simulink model "Simulation"  (R2026a)
settings: Solver=FixedStepAuto  StopTime=35  FixedStep=0.001  MaxStep=0.01  RelTol=1e-6
values from neighbouring files (symbols this model uses):
  a_max = 9.364072394    [params.m]    (also in scurve_test.m = 9.364)
  eta = 0.85    [params.m]
  j_max = 93.64072394    [params.m]
  K_aff = 0    [params.m]
  k_e = (V_max - (I_rated * R_m)) / omega_m    (= 0.0320704010623)    [params.m]
  k_t = tau_m / I_rated    (= 0.0381971863421)    [params.m]
  K_vff = 0    [params.m]
  L_m = 0.00147261    [params.m]
  N_total = N_gear * N_belt    (= 70)    [params.m]    (also in setup.m)
  q_final = 2*pi    (= 6.28318530718)    [params.m]
  q_init = 0    [params.m]
  R_m = 1.53982909    [params.m]
  v_max = 8.97597901    [params.m]
undefined symbols (not defined in the file or in its folder): X, Y, Z
libraries: sm_lib x16, nesl_utility x7, slpidlib x1
settings Model: Creator=thadzy  LastModifiedBy=thadzy
settings SimscapeCC: SimscapeNominalValues="[{\"value\":\"1\",\"unit\":\"A\"},{\"value\":\"1\",\"unit\":\"bar\"},{\"value\":\"1\",\"unit\":\"cm^2\"},{\"value\":\"1\",\"unit\":\"cm^3/s\"},{\"value\":\"1\",\"unit\":\"kJ/kg\"},{\"value\":\"1\",\"unit\":\"kW\"},{\"value\":\"1\",\"unit\":\"l\"},{\"value\":\"1\",\"unit\":\"N\"},{\"value\":\"1\",\"unit\":\"N*m\"},{\"value\":\"1\",\"unit\":\"V\"}]"  SimscapeLogType=none  SimscapeLogDataHistory=5000.0

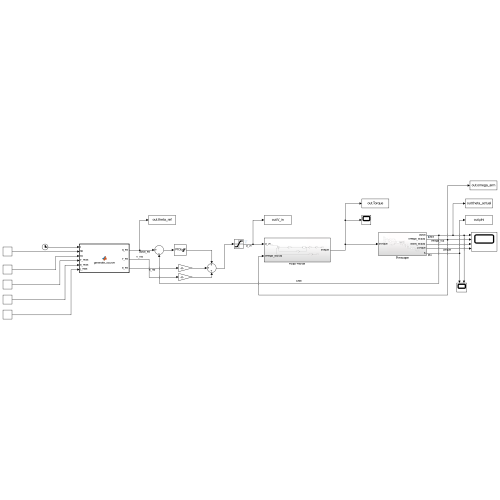
[thumbnail: Simulink's stored preview of the top-level diagram]
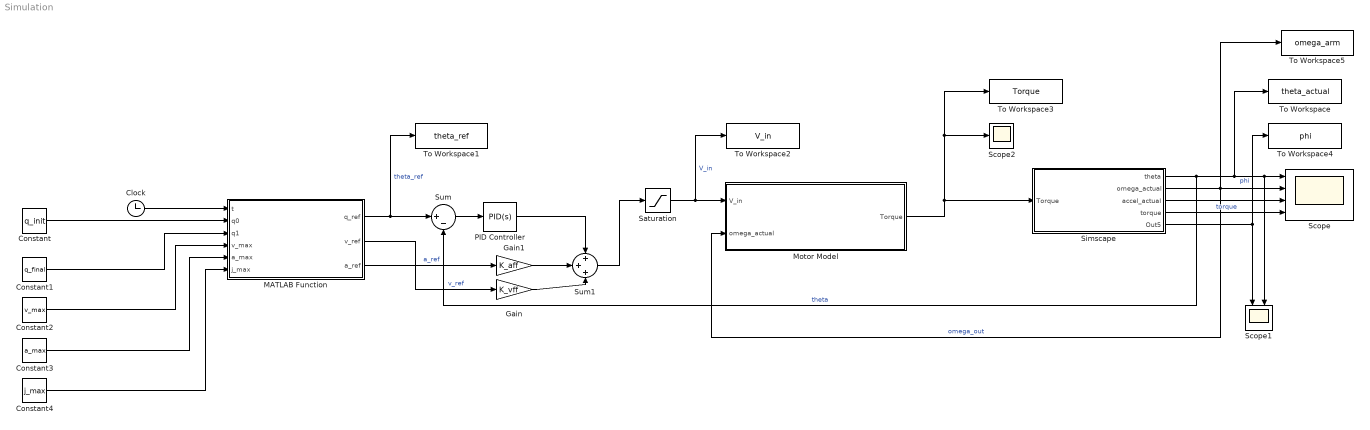
== system Simulation ==
  Clock : Clock
  Constant : Constant  Value=q_init
  Constant1 : Constant  Value=q_final
  Constant2 : Constant  Value=v_max
  Constant3 : Constant  Value=a_max
  Constant4 : Constant  Value=j_max
  Gain : Gain  Gain=K_vff
  Gain1 : Gain  Gain=K_aff
  MATLAB Function : MATLAB Function  TreatAsAtomicUnit=on
  Motor Model : Subsystem
  PID Controller : slpidlib/PID Controller  Controller=PID  Form=Parallel  TimeDomain=Continuous-time  UseExternalTs=off  SampleTime=-1  IntegratorMethod=Forward Euler  FilterMethod=Forward Euler  ControllerParametersSource=internal  P=1  I=0  UseKiTs=off  D=0.5  UseExternalDerivativeSource=off  N=200  UseFilter=on  TunerSelectOption=Transfer Function Based (PID Tuner App)  InitialConditionSource=internal  InitialConditionForIntegrator=0  InitialConditionForFilter=0  DifferentiatorICPrevScaledInput=0  ExternalReset=none  TrackingMode=off  Kt=1  LimitOutput=on  SatLimitsSource=internal  UpperSaturationLimit=24  LowerSaturationLimit=-24  LinearizeAsGain=on  AntiWindupMode=clamping  Kb=1  LimitIntegrator=off  UpperIntegratorSaturationLimit=inf  LowerIntegratorSaturationLimit=-inf  POutMin=[]  POutMax=[]  IOutMin=[]  IOutMax=[]  DOutMin=[]  DOutMax=[]  NOutMin=[]  NOutMax=[]  SumOutMin=[]  SumOutMax=[]  SaturationOutMin=[]  SaturationOutMax=[]  PParamMin=[]  PParamMax=[]  IParamMin=[]  IParamMax=[]  DParamMin=[]  DParamMax=[]  NParamMin=[]  NParamMax=[]  KbParamMin=[]  KbParamMax=[]  KtParamMin=[]  KtParamMax=[]  KbOutMin=[]  KbOutMax=[]  KtOutMin=[]  KtOutMax=[]  IntegratorOutMin=[]  IntegratorOutMax=[]  FilterOutMin=[]  FilterOutMax=[]  SumI1OutMin=[]  SumI1OutMax=[]  SumI2OutMin=[]  SumI2OutMax=[]  SumI3OutMin=[]  SumI3OutMax=[]  SumI4OutMin=[]  SumI4OutMax=[]  SumDOutMin=[]  SumDOutMax=[]  DifferentiatorOutMin=[]  DifferentiatorOutMax=[]  FilterDiffOutCoefMin=[]  FilterDiffOutCoefMax=[]  ReciprocalOutMin=[]  ReciprocalOutMax=[]  SumDenOutMin=[]  SumDenOutMax=[]  SumNumOutMin=[]  SumNumOutMax=[]  DivideOutMin=[]  DivideOutMax=[]  UdiffTsProdOutMin=[]  UdiffTsProdOutMax=[]  NTsProdOutMin=[]  NTsProdOutMax=[]  UintegralTsProdOutMin=[]  UintegralTsProdOutMax=[]  UngainTsProdOutMin=[]  UngainTsProdOutMax=[]  ClampingZeroOutDataTypeStr=Inherit: Inherit via back propagation  ClampingZeroOutMin=[]  ClampingZeroOutMax=[]  FilterDenConstantOutDataTypeStr=Inherit: Inherit via back propagation  FilterDenConstantOutMin=[]  FilterDenConstantOutMax=[]  PCopyOutDataTypeStr=Inherit: Inherit via back propagation  PCopyOutMin=[]  PCopyOutMax=[]  NCopyOutDataTypeStr=Inherit: Inherit via back propagation  NCopyOutMin=[]  NCopyOutMax=[]  IntegratorContinuousStateAttributes=''  IntegratorStateMustResolveToSignalObject=off  IntegratorRTWStateStorageClass=Auto  FilterContinuousStateAttributes=''  FilterStateMustResolveToSignalObject=off  FilterRTWStateStorageClass=Auto  ParallelPVariant=InternalParameters  IdealPVariant=Disabled  IVariant=InternalParameters  DVariant=InternalParameters  IntegratorVariant=Continuous  SatVariant=Enabled  AWVariant=ContClampingParallel  PCopyVariant=Disabled  TRVariant=Disabled  FdbkBlocksVariant=Forward  IdealPFdbkVariant=Disabled  SatFdbkVariant=Disabled  DerivativeFilterVariant=ContFilter  NVariant=InternalParameters  NCopyVariant=Disabled  FilterICVariant=InternalICsFilter  IntegratorICVariant=InternalICs  ExternalResetVariant=Disabled  TRSumVariant=Passthrough  SumFdbkVariant=Disabled  SumVariant=Sum_PID  TsampFilterVariant=InternalTs  TsampNgainVariant=Passthrough  TsampIntegralVariant=Disabled_SignalSpec  ExternalSaturationOutDataTypeStr=Inherit: Same as second input  DerivativeSourceVariant=ErrorSignal  PreIntVariant=InternalPreInt
  Saturation : Saturate  UpperLimit=24  LowerLimit=-24
  Scope : Scope  NumInputPorts=4
      settings: ActiveDisplayYMinimum=-23.989705041384052  ActiveDisplayYMaximum=22.744388235078567
  Scope1 : Scope  NumInputPorts=2
      settings: ActiveDisplayYMinimum=-16.623926963766117  ActiveDisplayYMaximum=10.381312120570854
  Scope2 : Scope
      settings: ActiveDisplayYMinimum=-0.24844726502323963  ActiveDisplayYMaximum=0.27894907226779375  DataLoggingVariableName=ScopeData2
  Simscape : Subsystem
  Sum : Sum  Inputs=|+-
  Sum1 : Sum  Inputs=+++
  To Workspace : ToWorkspace  VariableName=theta_actual  SaveFormat=Timeseries  SampleTime=-1
  To Workspace1 : ToWorkspace  VariableName=theta_ref  SaveFormat=Timeseries  SampleTime=-1
  To Workspace2 : ToWorkspace  VariableName=V_in  SaveFormat=Timeseries  SampleTime=-1
  To Workspace3 : ToWorkspace  VariableName=Torque  SaveFormat=Timeseries  SampleTime=-1
  To Workspace4 : ToWorkspace  VariableName=phi  SaveFormat=Timeseries  SampleTime=-1
  To Workspace5 : ToWorkspace  VariableName=omega_arm  SaveFormat=Timeseries  SampleTime=-1
  wires:
  Simscape/1(theta) -> To Workspace/1, Scope1/2, Scope/1, Sum/2  "theta"
  Simscape/2(omega_actual) -> To Workspace5/1, Scope/2, Motor Model/2(omega_actual)  "omega_out"
  Simscape/3(accel_actual) -> Scope/3
  Simscape/4(torque) -> Scope/4  "torque"
  Simscape/5(Out5) -> To Workspace4/1, Scope1/1  "phi"
  Motor Model/1(Torque) -> To Workspace3/1, Scope2/1, Simscape/1(Torque)
  Clock/1 -> MATLAB Function/1(t)
  MATLAB Function/1(q_ref) -> To Workspace1/1, Sum/1  "theta_ref"
  Constant/1 -> MATLAB Function/2(q0)
  Constant1/1 -> MATLAB Function/3(q1)
  Constant2/1 -> MATLAB Function/4(v_max)
  Constant3/1 -> MATLAB Function/5(a_max)
  Constant4/1 -> MATLAB Function/6(j_max)
  Sum/1 -> PID Controller/1
  MATLAB Function/2(v_ref) -> Gain/1  "v_ref"
  MATLAB Function/3(a_ref) -> Gain1/1  "a_ref"
  PID Controller/1 -> Sum1/1
  Gain1/1 -> Sum1/2
  Gain/1 -> Sum1/3
  Sum1/1 -> Saturation/1
  Saturation/1 -> To Workspace2/1, Motor Model/1(V_in)  "V_in"

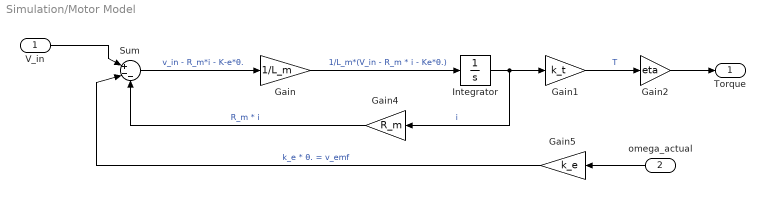
== system Simulation/Motor Model ==
  V_in : Inport
  omega_actual : Inport  Port=2
  Gain : Gain  Gain=1/L_m
  Gain1 : Gain  Gain=k_t
  Gain2 : Gain  Gain=eta
  Gain4 : Gain  Gain=R_m
  Gain5 : Gain  Gain=k_e
  Integrator : Integrator
  Sum : Sum  Inputs=|+--
  Torque : Outport
  wires:
  Gain/1 -> Integrator/1  "1/L_m*(V_in - R_m * i - Ke*θ.)"
  Gain5/1 -> Sum/2  "k_e * θ. = v_emf"
  Integrator/1 -> Gain4/1, Gain1/1  "i"
  V_in/1 -> Sum/1
  Sum/1 -> Gain/1  "v_in - R_m*i - K-e*θ."
  Gain4/1 -> Sum/3  "R_m * i"
  omega_actual/1 -> Gain5/1
  Gain1/1 -> Gain2/1  "T"
  Gain2/1 -> Torque/1

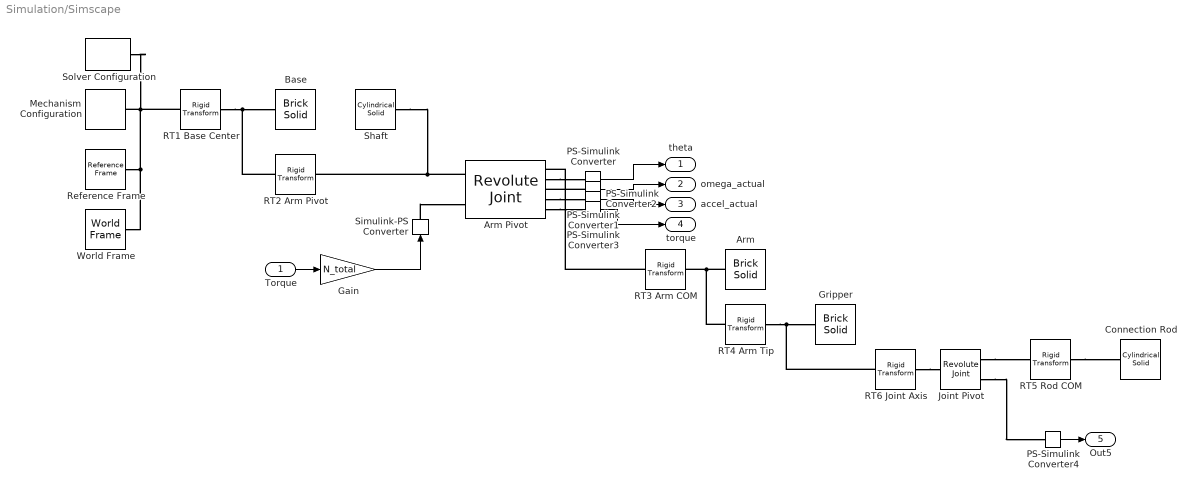
== system Simulation/Simscape ==
  Torque : Inport
  Arm : sm_lib/Body Elements/Brick Solid  BrickDimensions=[0.5 0.025 0.025]  BrickDimensionsUnits=m  ExportEntireGeometry=off  InertiaType=Custom  BasedOnType=Density  Density=2621  DensityUnits=kg/m^3  Mass=0.75357  MassUnits=kg  CenterOfMass=[0 0 0]  CenterOfMassUnits=m  MomentsOfInertia=[0.013479, 0.000131, 0.013479]  MomentsOfInertiaUnits=kg*m^2  ProductsOfInertia=[0, 0, -9.26e-6]  ProductsOfInertiaUnits=kg*m^2  GraphicType=FromGeometry  MarkerShape=Sphere  MarkerSize=10  GraphicVisPropType=SimpleVisualProperties  GraphicDiffuseColor=[0.4941 0.4941 0.502]  GraphicOpacity=1  GraphicSpecularColor=[0.5 0.5 0.5 1.0]  GraphicAmbientColor=[0.15 0.15 0.15 1.0]  GraphicEmissiveColor=[0.0 0.0 0.0 1.0]  GraphicShininess=75  DoExposeReferenceFrame=on  SerializedFrames=<Frames/>
  Arm Pivot : sm_lib/Joints/Revolute Joint  JointMode=Normal  CompositeWrenchDir=FollowerOnBase  CompositeWrenchFrame=BaseFrame  SenseConstraintForce=off  SenseConstraintTorque=off  SenseTotalForce=off  SenseTotalTorque=off  PositionTargetSpecify=off  PositionTargetPriority=High  PositionTargetValue=0  PositionTargetValueUnits=deg  VelocityTargetSpecify=off  VelocityTargetPriority=High  VelocityTargetValue=0  VelocityTargetValueUnits=deg/s  EquilibriumPosition=0  EquilibriumPositionUnits=deg  SpringStiffness=0  SpringStiffnessUnits=N*m/deg  DampingCoefficient=B_arm  DampingCoefficientUnits=N*m/(rad/s)  LowerLimitSpecify=off  LowerLimitBound=-90  LowerLimitBoundUnits=deg  LowerLimitStiffness=1e4  LowerLimitStiffnessUnits=N*m/deg  LowerLimitDamping=10  LowerLimitDampingUnits=N*m/(deg/s)  LowerLimitTransitionRegionWidth=0.1  LowerLimitTransitionRegionWidthUnits=deg  UpperLimitSpecify=off  UpperLimitBound=90  UpperLimitBoundUnits=deg  UpperLimitStiffness=1e4  UpperLimitStiffnessUnits=N*m/deg  UpperLimitDamping=10  UpperLimitDampingUnits=N*m/(deg/s)  UpperLimitTransitionRegionWidth=0.1  UpperLimitTransitionRegionWidthUnits=deg  TorqueActuationMode=InputTorque  MotionActuationMode=ComputedMotion  SensePosition=on  SenseVelocity=on  SenseAcceleration=on  SenseTorqueForce=on  SenseLowerLimitTorqueForce=off  SenseUpperLimitTorqueForce=off
  Base : sm_lib/Body Elements/Brick Solid  BrickDimensions=[0.16 0.16 0.15]  BrickDimensionsUnits=m  ExportEntireGeometry=off  InertiaType=CalculateFromGeometry  BasedOnType=Density  Density=2700  DensityUnits=kg/m^3  Mass=1  MassUnits=kg  CenterOfMass=[0 0 0]  CenterOfMassUnits=m  MomentsOfInertia=[1 1 1]  MomentsOfInertiaUnits=kg*m^2  ProductsOfInertia=[0 0 0]  ProductsOfInertiaUnits=kg*m^2  GraphicType=FromGeometry  MarkerShape=Sphere  MarkerSize=10  GraphicVisPropType=SimpleVisualProperties  GraphicDiffuseColor=[0.02745 0 1]  GraphicOpacity=1  GraphicSpecularColor=[0.5 0.5 0.5 1.0]  GraphicAmbientColor=[0.15 0.15 0.15 1.0]  GraphicEmissiveColor=[0.0 0.0 0.0 1.0]  GraphicShininess=75  DoExposeReferenceFrame=on  SerializedFrames=<Frames/>
  Connection Rod : sm_lib/Body Elements/Cylindrical Solid  CylinderRadius=0.005  CylinderRadiusUnits=m  CylinderLength=0.1  CylinderLengthUnits=m  ExportEntireGeometry=off  InertiaType=Custom  BasedOnType=Density  Density=7850  DensityUnits=kg/m^3  Mass=0.16408  MassUnits=kg  CenterOfMass=[0 0 0]  CenterOfMassUnits=m  MomentsOfInertia=[0.000169, 0.000152, 2.42e-5]  MomentsOfInertiaUnits=kg*m^2  ProductsOfInertia=[0 0 0]  ProductsOfInertiaUnits=kg*m^2  GraphicType=FromGeometry  MarkerShape=Sphere  MarkerSize=10  GraphicVisPropType=SimpleVisualProperties  GraphicDiffuseColor=[1 0 0.02745]  GraphicOpacity=1  GraphicSpecularColor=[0.5 0.5 0.5 1.0]  GraphicAmbientColor=[0.15 0.15 0.15 1.0]  GraphicEmissiveColor=[0.0 0.0 0.0 1.0]  GraphicShininess=75  DoExposeReferenceFrame=on  SerializedFrames=<Frames/>
  Gain : Gain  Gain=N_total
  Gripper : sm_lib/Body Elements/Brick Solid  BrickDimensions=[0.04 0.04 0.04]  BrickDimensionsUnits=m  ExportEntireGeometry=off  InertiaType=Custom  BasedOnType=Density  Density=1000  DensityUnits=kg/m^3  Mass=0.73897  MassUnits=kg  CenterOfMass=[0 0 0]  CenterOfMassUnits=m  MomentsOfInertia=[0.001819, 0.001273, 0.000760]  MomentsOfInertiaUnits=kg*m^2  ProductsOfInertia=[-8.41e-5, -6.54e-6, 9.06e-7]  ProductsOfInertiaUnits=kg*m^2  GraphicType=FromGeometry  MarkerShape=Sphere  MarkerSize=10  GraphicVisPropType=SimpleVisualProperties  GraphicDiffuseColor=[0.0902 1 0]  GraphicOpacity=1  GraphicSpecularColor=[0.5 0.5 0.5 1.0]  GraphicAmbientColor=[0.15 0.15 0.15 1.0]  GraphicEmissiveColor=[0.0 0.0 0.0 1.0]  GraphicShininess=75  DoExposeReferenceFrame=on  SerializedFrames=<Frames/>
  Joint Pivot : sm_lib/Joints/Revolute Joint  JointMode=Normal  CompositeWrenchDir=FollowerOnBase  CompositeWrenchFrame=BaseFrame  SenseConstraintForce=off  SenseConstraintTorque=off  SenseTotalForce=off  SenseTotalTorque=off  PositionTargetSpecify=off  PositionTargetPriority=High  PositionTargetValue=20  PositionTargetValueUnits=deg  VelocityTargetSpecify=off  VelocityTargetPriority=High  VelocityTargetValue=0  VelocityTargetValueUnits=deg/s  EquilibriumPosition=0  EquilibriumPositionUnits=deg  SpringStiffness=0  SpringStiffnessUnits=N*m/deg  DampingCoefficient=0.0006712  DampingCoefficientUnits=N*m/(rad/s)  LowerLimitSpecify=off  LowerLimitBound=-90  LowerLimitBoundUnits=deg  LowerLimitStiffness=1e4  LowerLimitStiffnessUnits=N*m/deg  LowerLimitDamping=10  LowerLimitDampingUnits=N*m/(deg/s)  LowerLimitTransitionRegionWidth=0.1  LowerLimitTransitionRegionWidthUnits=deg  UpperLimitSpecify=off  UpperLimitBound=90  UpperLimitBoundUnits=deg  UpperLimitStiffness=1e4  UpperLimitStiffnessUnits=N*m/deg  UpperLimitDamping=10  UpperLimitDampingUnits=N*m/(deg/s)  UpperLimitTransitionRegionWidth=0.1  UpperLimitTransitionRegionWidthUnits=deg  TorqueActuationMode=NoTorque  MotionActuationMode=ComputedMotion  SensePosition=on  SenseVelocity=off  SenseAcceleration=off  SenseTorqueForce=off  SenseLowerLimitTorqueForce=off  SenseUpperLimitTorqueForce=off
  Mechanism Configuration : sm_lib/Utilities/Mechanism Configuration  UniformGravity=Constant  GravityVector=[0 0 -9.80665]  GravityVectorUnits=m/s^2  LinearizationDelta=0.001  JointModeTransitionNonlinearIterations=2
  PS-Simulink Converter : nesl_utility/PS-Simulink Converter  PhysicalDomain=network_engine_domain  SubClassName=ps_output  LeftPortType=input  RightPortType=output  PseudoPeriodic=off  Frequencies=[]  VectorFormat=inherit  Unit=rad  AffineConversion=off
  PS-Simulink Converter1 : nesl_utility/PS-Simulink Converter  PhysicalDomain=network_engine_domain  SubClassName=ps_output  LeftPortType=input  RightPortType=output  PseudoPeriodic=off  Frequencies=[]  VectorFormat=inherit  Unit=rad/s  AffineConversion=off
  PS-Simulink Converter2 : nesl_utility/PS-Simulink Converter  PhysicalDomain=network_engine_domain  SubClassName=ps_output  LeftPortType=input  RightPortType=output  PseudoPeriodic=off  Frequencies=[]  VectorFormat=inherit  Unit=rad/s^2  AffineConversion=off
  PS-Simulink Converter3 : nesl_utility/PS-Simulink Converter  PhysicalDomain=network_engine_domain  SubClassName=ps_output  LeftPortType=input  RightPortType=output  PseudoPeriodic=off  Frequencies=[]  VectorFormat=inherit  Unit=N*m  AffineConversion=off
  PS-Simulink Converter4 : nesl_utility/PS-Simulink Converter  PhysicalDomain=network_engine_domain  SubClassName=ps_output  LeftPortType=input  RightPortType=output  PseudoPeriodic=off  Frequencies=[]  VectorFormat=inherit  Unit=rad  AffineConversion=off
  RT1 Base Center : sm_lib/Frames and Transforms/Rigid Transform  RotationMethod=None  FollAlignAxisA=+X  BaseAlignAxisA=+Y  FollAlignAxisB=+Y  BaseAlignAxisB=+Z  RotationStandardAxis=+Z  RotationAngle=0  RotationAngleUnits=deg  RotationArbitraryAxis=[0 0 1]  RotationSequenceAxes=FollowerAxes  RotationSequence=XYX  RotationSequenceAngles=[0 0 0]  RotationSequenceAnglesUnits=deg  RotationMatrix=[1 0 0;0 1 0;0 0 1]  Quaternion=[1 0 0 0]  TranslationMethod=Cartesian  TranslationCartesianOffset=[0, 0, 0.075]  TranslationCartesianOffsetUnits=m  TranslationStandardAxis=+Z  TranslationStandardOffset=0  TranslationStandardOffsetUnits=m  TranslationROffset=0  TranslationROffsetUnits=m  TranslationThetaOffset=0  TranslationThetaOffsetUnits=deg  TranslationZOffset=0  TranslationZOffsetUnits=m
  RT2 Arm Pivot : sm_lib/Frames and Transforms/Rigid Transform  RotationMethod=None  FollAlignAxisA=+X  BaseAlignAxisA=+Y  FollAlignAxisB=+Y  BaseAlignAxisB=+Z  RotationStandardAxis=+Z  RotationAngle=0  RotationAngleUnits=deg  RotationArbitraryAxis=[0 0 1]  RotationSequenceAxes=FollowerAxes  RotationSequence=XYX  RotationSequenceAngles=[0 0 0]  RotationSequenceAnglesUnits=deg  RotationMatrix=[1 0 0;0 1 0;0 0 1]  Quaternion=[1 0 0 0]  TranslationMethod=Cartesian  TranslationCartesianOffset=[0, 0, 0.075]  TranslationCartesianOffsetUnits=m  TranslationStandardAxis=+Z  TranslationStandardOffset=0  TranslationStandardOffsetUnits=m  TranslationROffset=0  TranslationROffsetUnits=m  TranslationThetaOffset=0  TranslationThetaOffsetUnits=deg  TranslationZOffset=0  TranslationZOffsetUnits=m
  RT3 Arm COM : sm_lib/Frames and Transforms/Rigid Transform  RotationMethod=None  FollAlignAxisA=+X  BaseAlignAxisA=+Y  FollAlignAxisB=+Y  BaseAlignAxisB=+Z  RotationStandardAxis=+Z  RotationAngle=0  RotationAngleUnits=deg  RotationArbitraryAxis=[0 0 1]  RotationSequenceAxes=FollowerAxes  RotationSequence=XYX  RotationSequenceAngles=[0 0 0]  RotationSequenceAnglesUnits=deg  RotationMatrix=[1 0 0;0 1 0;0 0 1]  Quaternion=[1 0 0 0]  TranslationMethod=Cartesian  TranslationCartesianOffset=[0.25, 0, 0]  TranslationCartesianOffsetUnits=m  TranslationStandardAxis=+Z  TranslationStandardOffset=0  TranslationStandardOffsetUnits=m  TranslationROffset=0  TranslationROffsetUnits=m  TranslationThetaOffset=0  TranslationThetaOffsetUnits=deg  TranslationZOffset=0  TranslationZOffsetUnits=m
  RT4 Arm Tip : sm_lib/Frames and Transforms/Rigid Transform  RotationMethod=None  FollAlignAxisA=+X  BaseAlignAxisA=+Y  FollAlignAxisB=+Y  BaseAlignAxisB=+Z  RotationStandardAxis=+Y  RotationAngle=90  RotationAngleUnits=deg  RotationArbitraryAxis=[0 0 1]  RotationSequenceAxes=FollowerAxes  RotationSequence=XYX  RotationSequenceAngles=[0 0 0]  RotationSequenceAnglesUnits=deg  RotationMatrix=[1 0 0;0 1 0;0 0 1]  Quaternion=[1 0 0 0]  TranslationMethod=Cartesian  TranslationCartesianOffset=[0.25, 0, 0]  TranslationCartesianOffsetUnits=m  TranslationStandardAxis=+Z  TranslationStandardOffset=0  TranslationStandardOffsetUnits=m  TranslationROffset=0  TranslationROffsetUnits=m  TranslationThetaOffset=0  TranslationThetaOffsetUnits=deg  TranslationZOffset=0  TranslationZOffsetUnits=m
  RT5 Rod COM : sm_lib/Frames and Transforms/Rigid Transform  RotationMethod=StandardAxis  FollAlignAxisA=+X  BaseAlignAxisA=+Y  FollAlignAxisB=+Y  BaseAlignAxisB=+Z  RotationStandardAxis=+X  RotationAngle=180  RotationAngleUnits=deg  RotationArbitraryAxis=[0 0 1]  RotationSequenceAxes=FollowerAxes  RotationSequence=XYZ  RotationSequenceAngles=[90, 0, 0]  RotationSequenceAnglesUnits=deg  RotationMatrix=[1 0 0;0 1 0;0 0 1]  Quaternion=[1 0 0 0]  TranslationMethod=Cartesian  TranslationCartesianOffset=[0, 0, -0.05]  TranslationCartesianOffsetUnits=m  TranslationStandardAxis=+Z  TranslationStandardOffset=0  TranslationStandardOffsetUnits=m  TranslationROffset=0  TranslationROffsetUnits=m  TranslationThetaOffset=0  TranslationThetaOffsetUnits=deg  TranslationZOffset=0  TranslationZOffsetUnits=m
  RT6 Joint Axis : sm_lib/Frames and Transforms/Rigid Transform  RotationMethod=None  FollAlignAxisA=+X  BaseAlignAxisA=+Y  FollAlignAxisB=+Y  BaseAlignAxisB=+Z  RotationStandardAxis=+X  RotationAngle=90  RotationAngleUnits=deg  RotationArbitraryAxis=[0 0 1]  RotationSequenceAxes=FollowerAxes  RotationSequence=XYZ  RotationSequenceAngles=[90, 0, 0]  RotationSequenceAnglesUnits=deg  RotationMatrix=[1 0 0;0 1 0;0 0 1]  Quaternion=[1 0 0 0]  TranslationMethod=Cartesian  TranslationCartesianOffset=[0, 0, 0]  TranslationCartesianOffsetUnits=m  TranslationStandardAxis=+Z  TranslationStandardOffset=0  TranslationStandardOffsetUnits=m  TranslationROffset=0  TranslationROffsetUnits=m  TranslationThetaOffset=0  TranslationThetaOffsetUnits=deg  TranslationZOffset=0  TranslationZOffsetUnits=m
  Reference Frame : sm_lib/Frames and Transforms/Reference Frame
  Shaft : sm_lib/Body Elements/Cylindrical Solid  CylinderRadius=0.0085  CylinderRadiusUnits=m  CylinderLength=0.03  CylinderLengthUnits=m  ExportEntireGeometry=off  InertiaType=CalculateFromGeometry  BasedOnType=Density  Density=7850  DensityUnits=kg/m^3  Mass=1  MassUnits=kg  CenterOfMass=[0 0 0]  CenterOfMassUnits=m  MomentsOfInertia=[1 1 1]  MomentsOfInertiaUnits=kg*m^2  ProductsOfInertia=[0 0 0]  ProductsOfInertiaUnits=kg*m^2  GraphicType=FromGeometry  MarkerShape=Sphere  MarkerSize=10  GraphicVisPropType=SimpleVisualProperties  GraphicDiffuseColor=[0.9961 0.9922 1]  GraphicOpacity=1  GraphicSpecularColor=[0.5 0.5 0.5 1.0]  GraphicAmbientColor=[0.15 0.15 0.15 1.0]  GraphicEmissiveColor=[0.0 0.0 0.0 1.0]  GraphicShininess=75  DoExposeReferenceFrame=on  SerializedFrames=<Frames/>
  Simulink-PS Converter : nesl_utility/Simulink-PS Converter  PhysicalDomain=network_engine_domain  SubClassName=ps_input  LeftPortType=input  RightPortType=output  PseudoPeriodic=off  Frequencies=[]  NoiseDistribution=none  NoiseParameters=[]  Unit=N*m  AffineConversion=off  FilteringAndDerivatives=provide  SimscapeFilterOrder=1  InputFilterTimeConstant=0.001  UdotUserProvided=0
  Solver Configuration : nesl_utility/Solver Configuration  PhysicalDomain=network_engine_domain  SubClassName=solver  LeftPortType=input  RightPortType=generic  Tones=[]  Harmonics=[]  SimulateNoise=off  Profile=off  UseLocalSampling=off  EnableSwitchedLinearOptims=on  FrequencyDomain=off  UseCCode=off  RelTol=0.001  AbsTol=0.001  MinStep=1e-09  ToWorkspace=off  RevertToSquareIcSolve=off  NumHomotopyIterations=100  PhasorMode=off  PhasorModeNumHarmonics=1  ConsistencySolver=NEWTON_XTOL_AFTER_FTOL  CanonicalOrdering=UNORDERED  OptimizeIntermediates=UNOPTIMIZED  IndexReductionMethod=DerivativeReplacement  DoDC=off  ResidualTolerance=1e-09  ConsistencyTolSource=GLOBAL  ConsistencyAbsTol=0.001  ConsistencyRelTol=0.001  ConsistencyTolFactor=0.001  UseLocalSolver=off  LocalSolverChoice=NE_BACKWARD_EULER_ADVANCER  ResolveIndetEquations=on  FunctionEvalNumThread=1  LocalSolverSampleTime=0.001  DoFixedCost=off  MaxNonlinIter=3  MaxModeIter=2  ComputeImpulses=off  ImpulseIterations=2  LinearAlgebra=auto  LinearAlgebraNumThread=0  EquationFormulation=NE_TIME_EF  DelaysMemoryBudget=1024  AutomaticFiltering=on  FilteringTimeConstant=0.001  PartitionStorageMethod=AS_NEEDED  PartitionMemoryBudget=1024  PartitionMethod=ROBUST  MultibodyUseLocalSolver=off  MultibodyLocalSolverChoice=ODE1  MultibodyLocalSolverSampleTime=0.001
  World Frame : sm_lib/Frames and Transforms/World Frame
  theta : Outport
  omega_actual : Outport  Port=2
  accel_actual : Outport  Port=3
  torque : Outport  Port=4
  Out5 : Outport  Port=5
  wires:
  PS-Simulink Converter1/1 -> omega_actual/1
  PS-Simulink Converter3/1 -> torque/1
  PS-Simulink Converter2/1 -> accel_actual/1
  PS-Simulink Converter/1 -> theta/1
  PS-Simulink Converter4/1 -> Out5/1
  Torque/1 -> Gain/1
  Gain/1 -> Simulink-PS Converter/1
  connections:
  RT4 Arm Tip/RConn1 -- RT6 Joint Axis/LConn1 -- Gripper/RConn1
  PS-Simulink Converter1/LConn1 -- Arm Pivot/RConn3
  Arm Pivot/RConn2 -- PS-Simulink Converter/LConn1
  Arm/RConn1 -- RT4 Arm Tip/LConn1 -- RT3 Arm COM/RConn1
  RT1 Base Center/RConn1 -- RT2 Arm Pivot/LConn1 -- Base/RConn1
  Arm Pivot/RConn5 -- PS-Simulink Converter3/LConn1
  Simulink-PS Converter/RConn1 -- Arm Pivot/LConn2
  Shaft/RConn1 -- Arm Pivot/LConn1 -- RT2 Arm Pivot/RConn1
  Arm Pivot/RConn4 -- PS-Simulink Converter2/LConn1
  Solver Configuration/RConn1 -- RT1 Base Center/LConn1 -- World Frame/RConn1 -- Reference Frame/RConn1 -- Mechanism Configuration/RConn1
  RT3 Arm COM/LConn1 -- Arm Pivot/RConn1
  Joint Pivot/RConn2 -- PS-Simulink Converter4/LConn1
  RT5 Rod COM/RConn1 -- Connection Rod/RConn1
  RT6 Joint Axis/RConn1 -- Joint Pivot/LConn1
  Joint Pivot/RConn1 -- RT5 Rod COM/LConn1

== matlab function Simulation/MATLAB Function ==
  data: t input; q_ref output; q0 input; q1 input; v_max input; a_max input; j_max input; v_ref output; a_ref output
% /**
%  * @function generate_scurve
%  * @description Generates a complete 7-segment jerk-limited S-Curve trajectory.
%  * @param {double} t - Current simulation time (s).
%  * @param {double} q0 - Initial position (rad).
%  * @param {double} q1 - Final target position (rad).
%  * @param {double} v_max - Maximum allowable velocity (rad/s).
%  * @param {double} a_max - Maximum allowable acceleration (rad/s^2).
%  * @param {double} j_max - Maximum allowable jerk (rad/s^3).
%  * @returns {double} q_ref - Reference position at time t.
%  * @returns {double} v_ref - Reference velocity at time t.
%  * @returns {double} a_ref - Reference acceleration at time t.
%  */
function [q_ref, v_ref, a_ref] = generate_scurve(t, q0, q1, v_max, a_max, j_max)
    
    % Calculate total displacement and phase durations
    h = q1 - q0;
    tj = a_max / j_max;
    ta = v_max / a_max;
    tv = (h / v_max) - ta;
    
    % Time breakpoints
    t1 = tj;
    t2 = ta;
    t3 = ta + tj;
    t4 = ta + tj + tv;
    t7 = t4 + ta + tj; % Total trajectory time
    
    % Initial conditions
    if t <= 0
        q_ref = q0; v_ref = 0; a_ref = 0;
        
    % Acceleration Phase (Segments 1 to 3)
    elseif t < t1
        % Segment 1: Jerk bounded acceleration
        a_ref = j_max * t;
        v_ref = 0.5 * j_max * t^2;
        q_ref = q0 + (1/6) * j_max * t^3;
        
    elseif t < t2
        % Segment 2: Constant acceleration
        dt = t - t1;
        a_ref = a_max;
        v_ref = (0.5 * j_max * t1^2) + a_max * dt;
        q_ref = q0 + (1/6) * j_max * t1^3 + (0.5 * j_max * t1^2) * dt + 0.5 * a_max * dt^2;
        
    elseif t < t3
        % Segment 3: Jerk bounded deceleration to reach constant velocity
        dt = t - t2;
        a_ref = a_max - j_max * dt;
        v2 = (0.5 * j_max * t1^2) + a_max * (t2 - t1);
        q2 = q0 + (1/6) * j_max * t1^3 + (0.5 * j_max * t1^2) * (t2 - t1) + 0.5 * a_max * (t2 - t1)^2;
        v_ref = v2 + a_max * dt - 0.5 * j_max * dt^2;
        q_ref = q2 + v2 * dt + 0.5 * a_max * dt^2 - (1/6) * j_max * dt^3;
        
    % Constant Velocity Phase (Segment 4)
    elseif t < t4
        dt = t - t3;
        a_ref = 0;
        v_ref = v_max;
        q3 = q0 + h/2 - v_max * (tv/2);
        q_ref = q3 + v_max * dt;
        
    % Deceleration Phase using time-reversal symmetry (Segments 5 to 7)
    elseif t < t7
        tau = t7 - t; % Time remaining
        
        if tau < t1
            % Equivalent to Segment 7
            a_ref = -j_max * tau;
            v_ref = 0.5 * j_max * tau^2;
            q_ref = q1 - (1/6) * j_max * tau^3;
            
        elseif tau < t2
            % Equivalent to Segment 6
            dt_tau = tau - t1;
            a_ref = -a_max;
            v_ref = (0.5 * j_max * t1^2) + a_max * dt_tau;
            q_ref = q1 - ((1/6) * j_max * t1^3 + (0.5 * j_max * t1^2) * dt_tau + 0.5 * a_max * dt_tau^2);
            
        else
            % Equivalent to Segment 5
            dt_tau = tau - t2;
            a_ref = -a_max + j_max * dt_tau;
            v2_tau = (0.5 * j_max * t1^2) + a_max * (t2 - t1);
            q2_tau = (1/6) * j_max * t1^3 + (0.5 * j_max * t1^2) * (t2 - t1) + 0.5 * a_max * (t2 - t1)^2;
            v_ref = v2_tau + a_max * dt_tau - 0.5 * j_max * dt_tau^2;
            q_ref = q1 - (q2_tau + v2_tau * dt_tau + 0.5 * a_max * dt_tau^2 - (1/6) * j_max * dt_tau^3);
        end
        
    % Final State Reached
    else
        q_ref = q1;
        v_ref = 0;
        a_ref = 0;
    end
end
